simulink model "full_adder"  (R2018b)
settings: Solver=VariableStepAuto  StartTime=0.0  StopTime=10.0  RelTol=1e-3
settings Model: Creator=Edoardo Debenedetti  LastModifiedBy=Edoardo
settings DebuggingCC: LibraryContextMissingDiagnostic=none
settings SFSimCC: SimUseLocalCustomCode=off
settings RTWCC: RTWUseLocalCustomCode=off

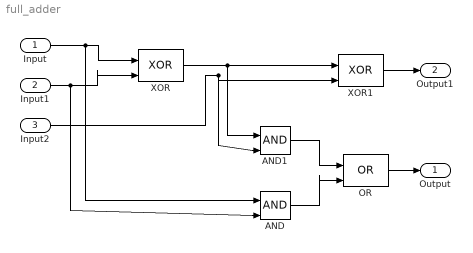
== system full_adder ==
  Input : Inport
  Input1 : Inport  Port=2
  Input2 : Inport  Port=3
  AND : Logic  IconShape=distinctive  AllPortsSameDT=off  OutDataTypeStr=boolean
  AND1 : Logic  IconShape=distinctive  AllPortsSameDT=off  OutDataTypeStr=boolean
  OR : Logic  Operator=OR  IconShape=distinctive  AllPortsSameDT=off  OutDataTypeStr=boolean
  XOR : Logic  Operator=XOR  IconShape=distinctive  AllPortsSameDT=off  OutDataTypeStr=boolean
  XOR1 : Logic  Operator=XOR  IconShape=distinctive  AllPortsSameDT=off  OutDataTypeStr=boolean
  Output : Outport
  Output1 : Outport  Port=2
  wires:
  Input/1 -> AND/1, XOR/1
  Input1/1 -> AND/2, XOR/2
  XOR/1 -> AND1/1, XOR1/1
  Input2/1 -> AND1/2, XOR1/2
  AND1/1 -> OR/1
  AND/1 -> OR/2
  OR/1 -> Output/1
  XOR1/1 -> Output1/1
